simulink model "ControlePD_ind_sat_itemb"  (R2018b)
settings: Solver=FixedStepAuto  StartTime=0.0  StopTime=9  FixedStep=1/100  RelTol=1e-3
values from neighbouring files (symbols this model uses):
  Beff = 50    [Ex5.m]
  Jeff = 2.2    [Ex5.m]
  K = 17.7    [Ex5.m]
  Kd = (2*qsi*wn*Jeff - Beff)/K    (= -0.338983050847)    [Ex5.m]
  Kp = (wn^2*Jeff)/K    (= 12.4293785311)    [Ex5.m]
  N = 10    [Ex5.m]
  r = 1    [Ex5.m]
  SP_theta = ThetaA0    [Ex5.m]
undefined symbols (not defined in the file or in its folder): thpath
libraries: simulink x1
settings Model: Creator=Karoline  LastModifiedBy=Karoline
settings SFSimCC: SimUseLocalCustomCode=off
settings RTWCC: RTWUseLocalCustomCode=off
settings CodeAppCC: StateflowObjectComments=on

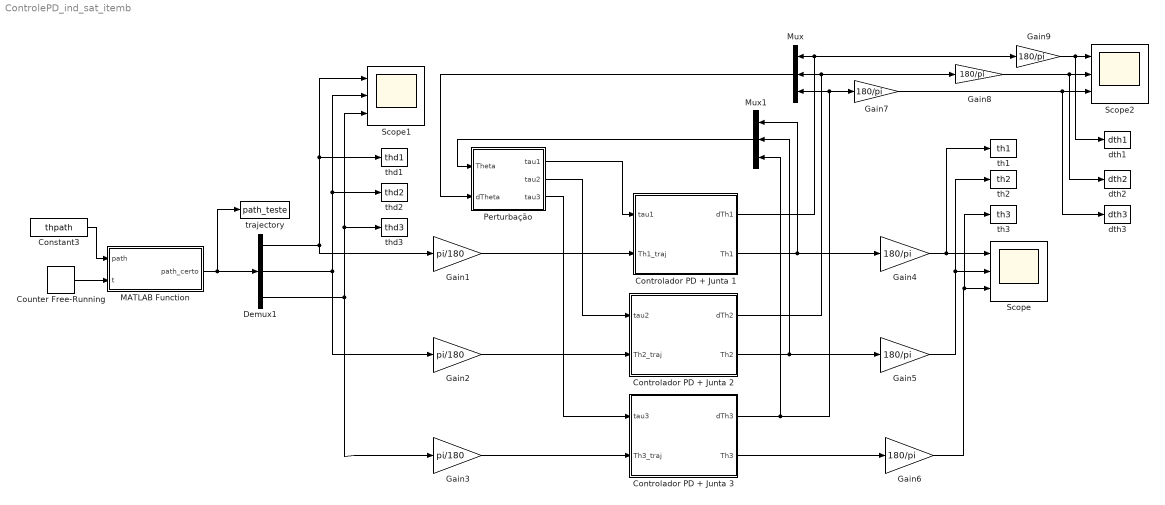
== system ControlePD_ind_sat_itemb ==
  Constant3 : Constant  Value=thpath
  Controlador PD + Junta 1 : Subsystem
  Controlador PD + Junta 2 : Subsystem
  Controlador PD + Junta 3 : Subsystem
  Counter Free-Running : simulink/Sources/Counter Free-Running  NumBits=16  tsamp=1/100
  Demux1 : Demux  Outputs=3
  Gain1 : Gain  Gain=pi/180
  Gain2 : Gain  Gain=pi/180
  Gain3 : Gain  Gain=pi/180
  Gain{4..9} (6 alike) : Gain  Gain=180/pi
  MATLAB Function : MATLAB Function  TreatAsAtomicUnit=on
  Mux : Mux  Inputs=3
  Mux1 : Mux  Inputs=3
  Perturbação : Subsystem
  Scope : Scope  NumInputPorts=3
  Scope1 : Scope  NumInputPorts=3
  Scope2 : Scope  NumInputPorts=3
  dth1 : ToWorkspace  VariableName=dth1  SampleTime=-1
  dth2 : ToWorkspace  VariableName=dth2  SampleTime=-1
  dth3 : ToWorkspace  VariableName=dth3  SampleTime=-1
  th1 : ToWorkspace  VariableName=th1  SampleTime=-1
  th2 : ToWorkspace  VariableName=th2  SampleTime=-1
  th3 : ToWorkspace  VariableName=th3  SampleTime=-1
  "thd1 " : ToWorkspace  VariableName=thd1  SampleTime=-1
  "thd2 " : ToWorkspace  VariableName=thd2  SampleTime=-1
  thd3 : ToWorkspace  VariableName=thd3  SampleTime=-1
  trajectory : ToWorkspace  VariableName=path_teste  SampleTime=-1
  wires:
  Demux1/1 -> Gain1/1, Scope1/1, "thd1 "/1
  Perturbação/1(tau1) -> Controlador PD + Junta 1/1(tau1)
  Mux/1 -> Perturbação/2(dTheta)
  Mux1/1 -> Perturbação/1(Theta)
  Demux1/3 -> Gain3/1, Scope1/3, thd3/1
  Demux1/2 -> Gain2/1, Scope1/2, "thd2 "/1
  Gain1/1 -> Controlador PD + Junta 1/2(Th1_traj)
  Gain2/1 -> Controlador PD + Junta 2/2(Th2_traj)
  Gain3/1 -> Controlador PD + Junta 3/2(Th3_traj)
  Gain4/1 -> th1/1, Scope/1
  Gain5/1 -> th2/1, Scope/2
  Gain6/1 -> th3/1, Scope/3
  Controlador PD + Junta 1/1("dTh1 ") -> Mux/1, Gain9/1
  Controlador PD + Junta 2/1("dTh2 ") -> Mux/2, Gain8/1
  Controlador PD + Junta 3/1("dTh3 ") -> Mux1/3, Mux/3, Gain7/1
  Controlador PD + Junta 1/2(Th1) -> Mux1/1, Gain4/1
  Controlador PD + Junta 2/2(Th2) -> Mux1/2, Gain5/1
  Controlador PD + Junta 3/2(Th3) -> Gain6/1
  Perturbação/2(tau2) -> Controlador PD + Junta 2/1(tau2)
  Perturbação/3(tau3) -> Controlador PD + Junta 3/1(tau3)
  Gain7/1 -> dth3/1, Scope2/3
  Gain8/1 -> dth2/1, Scope2/2
  Gain9/1 -> dth1/1, Scope2/1
  Constant3/1 -> MATLAB Function/1(path)
  MATLAB Function/1(path_certo) -> trajectory/1, Demux1/1
  Counter Free-Running/1 -> MATLAB Function/2(t)

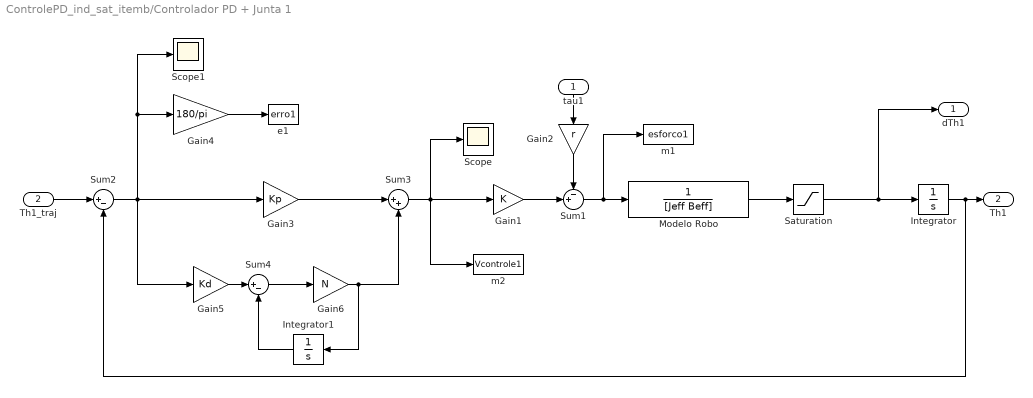
== system ControlePD_ind_sat_itemb/Controlador PD + Junta 1 ==
  tau1 : Inport
  Th1_traj : Inport  Port=2
  Gain1 : Gain  Gain=K
  Gain2 : Gain  Gain=r
  Gain3 : Gain  Gain=Kp
  Gain4 : Gain  Gain=180/pi
  Gain5 : Gain  Gain=Kd
  Gain6 : Gain  Gain=N
  Integrator : Integrator  InitialCondition=SP_theta(1)*pi/180
  Integrator1 : Integrator
  Modelo Robo : TransferFcn  Denominator=[Jeff Beff]
  Saturation : Saturate  UpperLimit=10*pi/180  LowerLimit=-10*pi/180
  Scope : Scope
  Scope1 : Scope
  Sum1 : Sum  Inputs=-+|
  Sum2 : Sum  Inputs=|+-
  Sum3 : Sum  Inputs=|++
  Sum4 : Sum  Inputs=|+-
  e1 : ToWorkspace  VariableName=erro1  SampleTime=-1
  m1 : ToWorkspace  VariableName=esforco1  SampleTime=-1
  m2 : ToWorkspace  VariableName=Vcontrole1  SampleTime=-1
  "dTh1 " : Outport
  Th1 : Outport  Port=2
  wires:
  tau1/1 -> Gain2/1
  Modelo Robo/1 -> Saturation/1
  Gain1/1 -> Sum1/2
  Sum1/1 -> m1/1, Modelo Robo/1
  Integrator/1 -> Th1/1, Sum2/2
  Th1_traj/1 -> Sum2/1
  Gain2/1 -> Sum1/1
  Sum2/1 -> Gain5/1, Gain3/1, Scope1/1, Gain4/1
  Gain4/1 -> e1/1
  Gain3/1 -> Sum3/1
  Gain5/1 -> Sum4/1
  Sum4/1 -> Gain6/1
  Gain6/1 -> Sum3/2, Integrator1/1
  Integrator1/1 -> Sum4/2
  Sum3/1 -> m2/1, Scope/1, Gain1/1
  Saturation/1 -> "dTh1 "/1, Integrator/1

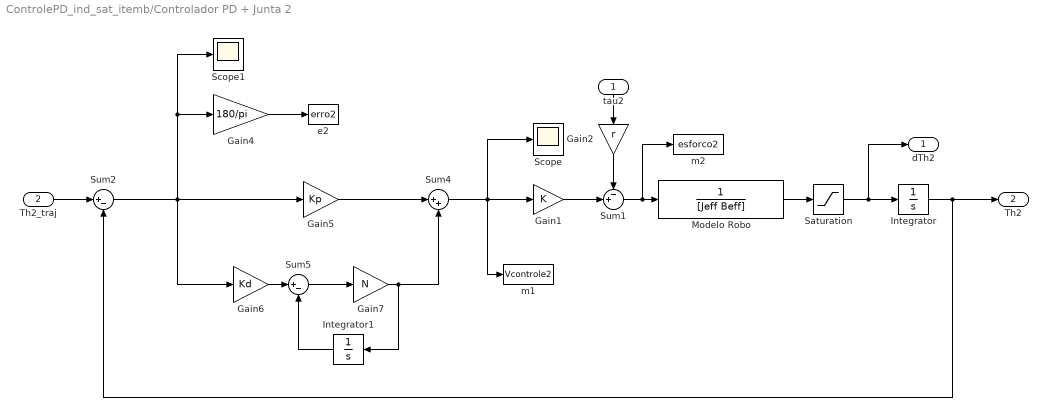
== system ControlePD_ind_sat_itemb/Controlador PD + Junta 2 ==
  tau2 : Inport
  Th2_traj : Inport  Port=2
  Gain1 : Gain  Gain=K
  Gain2 : Gain  Gain=r
  Gain4 : Gain  Gain=180/pi
  Gain5 : Gain  Gain=Kp
  Gain6 : Gain  Gain=Kd
  Gain7 : Gain  Gain=N
  Integrator : Integrator  InitialCondition=SP_theta(2)*pi/180
  Integrator1 : Integrator
  "Modelo Robo " : TransferFcn  Denominator=[Jeff Beff]
  Saturation : Saturate  UpperLimit=10*pi/180  LowerLimit=-10*pi/180
  Scope : Scope
  Scope1 : Scope
  Sum1 : Sum  Inputs=-+|
  Sum2 : Sum  Inputs=|+-
  Sum4 : Sum  Inputs=|++
  Sum5 : Sum  Inputs=|+-
  e2 : ToWorkspace  VariableName=erro2  SampleTime=-1
  m1 : ToWorkspace  VariableName=Vcontrole2  SampleTime=-1
  m2 : ToWorkspace  VariableName=esforco2  SampleTime=-1
  "dTh2 " : Outport
  Th2 : Outport  Port=2
  wires:
  tau2/1 -> Gain2/1
  "Modelo Robo "/1 -> Saturation/1
  Gain1/1 -> Sum1/2
  Sum1/1 -> m2/1, "Modelo Robo "/1
  Integrator/1 -> Th2/1, Sum2/2
  Th2_traj/1 -> Sum2/1
  Gain2/1 -> Sum1/1
  Gain4/1 -> e2/1
  Gain5/1 -> Sum4/1
  Sum2/1 -> Scope1/1, Gain4/1, Gain6/1, Gain5/1
  Integrator1/1 -> Sum5/2
  Sum5/1 -> Gain7/1
  Gain6/1 -> Sum5/1
  Gain7/1 -> Sum4/2, Integrator1/1
  Sum4/1 -> m1/1, Scope/1, Gain1/1
  Saturation/1 -> "dTh2 "/1, Integrator/1

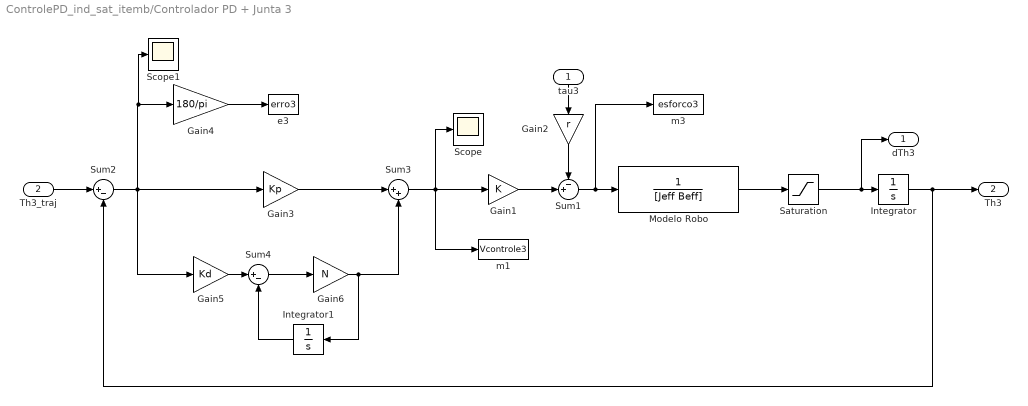
== system ControlePD_ind_sat_itemb/Controlador PD + Junta 3 ==
  tau3 : Inport
  Th3_traj : Inport  Port=2
  Gain1 : Gain  Gain=K
  Gain2 : Gain  Gain=r
  Gain3 : Gain  Gain=Kp
  Gain4 : Gain  Gain=180/pi
  Gain5 : Gain  Gain=Kd
  Gain6 : Gain  Gain=N
  Integrator : Integrator  InitialCondition=SP_theta(3)*pi/180
  Integrator1 : Integrator
  Modelo Robo : TransferFcn  Denominator=[Jeff Beff]
  Saturation : Saturate  UpperLimit=10*pi/180  LowerLimit=-10*pi/180
  Scope : Scope
  Scope1 : Scope
  Sum1 : Sum  Inputs=-+|
  Sum2 : Sum  Inputs=|+-
  Sum3 : Sum  Inputs=|++
  Sum4 : Sum  Inputs=|+-
  e3 : ToWorkspace  VariableName=erro3  SampleTime=-1
  m1 : ToWorkspace  VariableName=Vcontrole3  SampleTime=-1
  m3 : ToWorkspace  VariableName=esforco3  SampleTime=-1
  "dTh3 " : Outport
  Th3 : Outport  Port=2
  wires:
  tau3/1 -> Gain2/1
  Modelo Robo/1 -> Saturation/1
  Gain1/1 -> Sum1/2
  Sum1/1 -> m3/1, Modelo Robo/1
  Integrator/1 -> Th3/1, Sum2/2
  Th3_traj/1 -> Sum2/1
  Gain2/1 -> Sum1/1
  Gain4/1 -> e3/1
  Gain3/1 -> Sum3/1
  Sum2/1 -> Scope1/1, Gain4/1, Gain5/1, Gain3/1
  Integrator1/1 -> Sum4/2
  Sum4/1 -> Gain6/1
  Gain5/1 -> Sum4/1
  Gain6/1 -> Sum3/2, Integrator1/1
  Sum3/1 -> m1/1, Scope/1, Gain1/1
  Saturation/1 -> Integrator/1, "dTh3 "/1

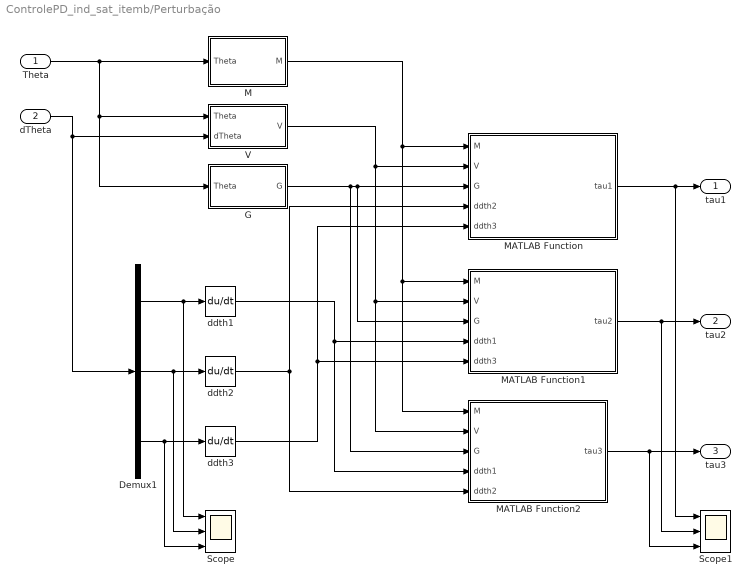
== system ControlePD_ind_sat_itemb/Perturbação ==
  Theta : Inport
  dTheta : Inport  Port=2
  Demux1 : Demux  Outputs=3
  G : Subsystem
  M : Subsystem
  MATLAB Function : MATLAB Function  TreatAsAtomicUnit=on
  MATLAB Function1 : MATLAB Function  TreatAsAtomicUnit=on
  MATLAB Function2 : MATLAB Function  TreatAsAtomicUnit=on
  Scope : Scope  NumInputPorts=3
  Scope1 : Scope  NumInputPorts=3
  V : Subsystem
  ddth1 : Derivative
  ddth2 : Derivative
  ddth3 : Derivative
  tau1 : Outport
  tau2 : Outport  Port=2
  tau3 : Outport  Port=3
  wires:
  dTheta/1 -> Demux1/1, V/2(dTheta)
  G/1(G) -> MATLAB Function2/3(G), MATLAB Function1/3(G), MATLAB Function/3(G)
  V/1(V) -> MATLAB Function/2(V), MATLAB Function1/2(V), MATLAB Function2/2(V)
  M/1(M) -> MATLAB Function2/1(M), MATLAB Function1/1(M), MATLAB Function/1(M)
  Theta/1 -> M/1(Theta), V/1(Theta), G/1(Theta)
  Demux1/1 -> Scope/1, ddth1/1
  Demux1/2 -> Scope/2, ddth2/1
  Demux1/3 -> Scope/3, ddth3/1
  ddth1/1 -> MATLAB Function2/4(ddth1), MATLAB Function1/4(ddth1)
  ddth3/1 -> MATLAB Function/5(ddth3), MATLAB Function1/5(ddth3)
  ddth2/1 -> MATLAB Function/4(ddth2), MATLAB Function2/5(ddth2)
  MATLAB Function/1(tau1) -> Scope1/1, tau1/1
  MATLAB Function1/1(tau2) -> Scope1/2, tau2/1
  MATLAB Function2/1(tau3) -> Scope1/3, tau3/1

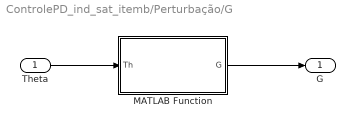
== system ControlePD_ind_sat_itemb/Perturbação/G ==
  Theta : Inport
  MATLAB Function : MATLAB Function  TreatAsAtomicUnit=on
  G : Outport
  wires:
  Theta/1 -> MATLAB Function/1(Th)
  MATLAB Function/1(G) -> G/1

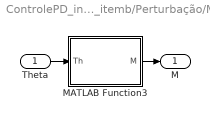
== system ControlePD_ind_sat_itemb/Perturbação/M ==
  Theta : Inport
  MATLAB Function3 : MATLAB Function  TreatAsAtomicUnit=on
  M : Outport
  wires:
  Theta/1 -> MATLAB Function3/1(Th)
  MATLAB Function3/1(M) -> M/1

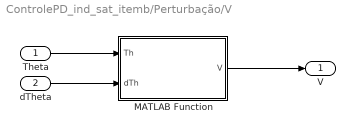
== system ControlePD_ind_sat_itemb/Perturbação/V ==
  Theta : Inport
  dTheta : Inport  Port=2
  MATLAB Function : MATLAB Function  TreatAsAtomicUnit=on
  V : Outport
  wires:
  Theta/1 -> MATLAB Function/1(Th)
  MATLAB Function/1(V) -> V/1
  dTheta/1 -> MATLAB Function/2(dTh)

== matlab function ControlePD_ind_sat_itemb/Perturbação/V/MATLAB Function ==
  data: Th input; V output; dTh input
function V = calcul_V(Th,dTh)

th1 = Th(1);
th2 = Th(2);
th3 = Th(3);

dth1 = dTh(1);
dth2 = dTh(2);
dth3 = dTh(3);

V =[-(33*dth2^2*sin(th2))/40 - (33*dth1*dth2*sin(th2))/20;...
    (33*dth1^2*sin(th2))/40;...
    0];

== matlab function ControlePD_ind_sat_itemb/Perturbação/G/MATLAB Function ==
  data: Th input; G output
function G = calcul_G(Th)

th1 = Th(1);
th2 = Th(2);
th3 = Th(3);

G = [(1617*cos(th1 + th2))/100 + (3871*cos(th1))/100;...
    (1617*cos(th1 + th2))/100;...
    0];

== matlab function ControlePD_ind_sat_itemb/Perturbação/MATLAB Function1 ==
  data: M input; V input; tau2 output; G input; ddth1 input; ddth3 input
function tau2  = calcul_dk2(M,V,G,ddth1, ddth3)


% tau2 = m21*ddth1 + m23*ddth3 + v2 + g2;
tau2 = M(2,1)*ddth1 + M(2,3)*ddth3 + V(2) + G(2);

== matlab function ControlePD_ind_sat_itemb/Perturbação/MATLAB Function ==
  data: M input; V input; tau1 output; G input; ddth2 input; ddth3 input
function tau1  = calcul_dk1(M,V,G,ddth2,ddth3)


% tau1 = m12*ddth2 + m13*ddth3 + v1 + g1;
tau1 = M(1,2)*ddth2 + M(1,3)*ddth3 + V(1) + G(1);

== matlab function ControlePD_ind_sat_itemb/Perturbação/MATLAB Function2 ==
  data: M input; V input; tau3 output; G input; ddth1 input; ddth2 input
function tau3  = calcul_dk3(M, V, G, ddth1, ddth2)



% tau3 = m31*ddth1 + m32*ddth2 + v3 + g3;
tau3 = M(3,1)*ddth1 + M(3,2)*ddth2 + V(3) + G(3);

== matlab function ControlePD_ind_sat_itemb/Perturbação/M/MATLAB Function3 ==
  data: Th input; M output
function M = calcul_M(Th)

th1 = Th(1);
th2 = Th(2);
th3 = Th(3);

M = [(33*cos(th2))/20 + 29/10, (33*cos(th2))/40 + 37/40, 1/10;...
     (33*cos(th2))/40 + 37/40,                    37/40, 1/10;...
                         1/10,                     1/10, 1/10];

== matlab function ControlePD_ind_sat_itemb/MATLAB Function ==
  data: path input; path_certo output; t input
function path_certo = fcn(path,t)
path_certo = path(t+1,:);
